simulink model "lateral_autopilot_2e"  (R2018b)
settings: Solver=VariableStepAuto  StartTime=0.0  StopTime=500  RelTol=1e-3
values from neighbouring files (symbols this model uses):
  A = [ ... (first row only)    [lateral_autopilot_2f_params.m]
  B = [0 0 0 0 7.5]'    [lateral_autopilot_2f_params.m]
  C = [eye(4) zeros(4,1)]    [lateral_autopilot_2f_params.m]
  d = 1.5    [lateral_autopilot_2d_params.m]    (also in lateral_autopilot_2f_params.m)
  g = 9.81    [lateral_autopilot_2d_params.m]    (also in lateral_autopilot_2f_params.m)
  kd_phi = (2*zeta_phi*omega_n_phi-a_phi_1)/a_phi_2    [lateral_autopilot_2d_params.m]    (also in lateral_autopilot_2f_params.m)
  ki_chi = omega_chi_phi^2*vg/g    [lateral_autopilot_2d_params.m]    (also in lateral_autopilot_2f_params.m)
  kp_chi = 2*zeta_chi*omega_chi_phi*vg/g    [lateral_autopilot_2d_params.m]    (also in lateral_autopilot_2f_params.m)
  kp_phi = (aileron_max/error_max)*sign(a_phi_2)    [lateral_autopilot_2d_params.m]    (also in lateral_autopilot_2f_params.m)
  vg = 580*km_h2m_s    (= 161.111111111)    [lateral_autopilot_2d_params.m]    (also in lateral_autopilot_2f_params.m)
libraries: simulink_extras x3, simulink x1
settings Model: Creator=dino  LastModifiedBy=dino

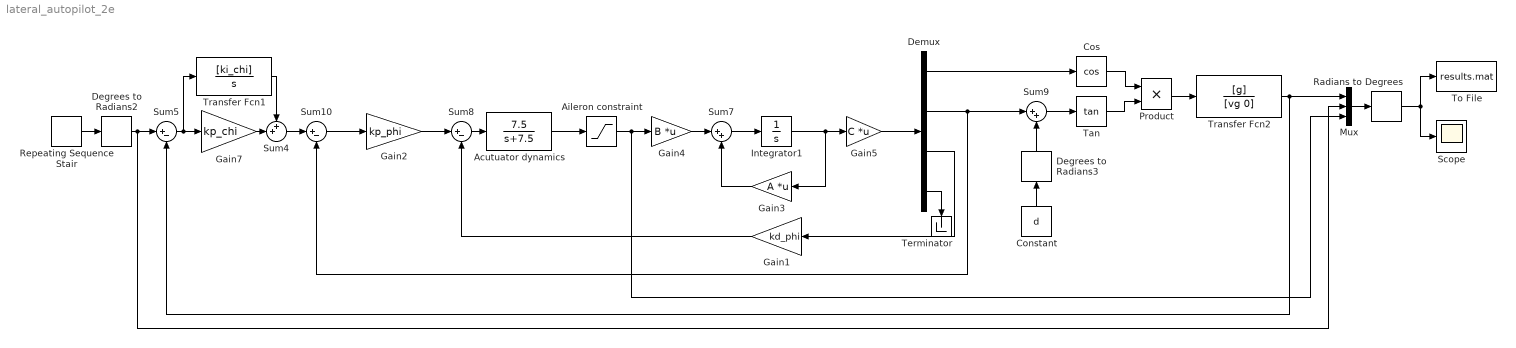
== system lateral_autopilot_2e ==
  Acutuator dynamics : TransferFcn  Numerator=[0 7.5]  Denominator=[1 7.5]
  "Aileron constraint " : Saturate  UpperLimit=30*deg2rad  LowerLimit=-30*deg2rad
  Constant : Constant  Value=d
  Cos : Trigonometry  Operator=cos
  Degrees to Radians2 : simulink_extras/Transformations/Degrees to Radians
  Degrees to Radians3 : simulink_extras/Transformations/Degrees to Radians
  Demux : Demux
  Gain1 : Gain  Gain=kd_phi
  Gain2 : Gain  Gain=kp_phi
  Gain3 : Gain  Gain=A  Multiplication=Matrix(K*u)
  Gain4 : Gain  Gain=B  Multiplication=Matrix(K*u)
  Gain5 : Gain  Gain=C  Multiplication=Matrix(K*u)
  Gain7 : Gain  Gain=kp_chi
  Integrator1 : Integrator
  Mux : Mux  Inputs=3
  Product : Product
  Radians to Degrees : simulink_extras/Transformations/Radians to Degrees
  Repeating Sequence Stair : simulink/Sources/Repeating Sequence Stair  OutValues=step_series.'  tsamp=60  OutMin=[]  OutMax=[]  OutDataTypeStr=double  OutputDataTypeScalingMode=double  OutDataType=fixdt(0,8)  ConRadixGroup=Best Precision: Vector-wise  OutScaling=2^-12
  Scope : Scope
  Sum10 : Sum  Inputs=|+-
  Sum4 : Sum  Inputs=++|
  Sum5 : Sum  Inputs=|+-
  Sum7 : Sum  Inputs=|++
  Sum8 : Sum  Inputs=|+-
  Sum9 : Sum  Inputs=|++
  Tan : Trigonometry  Operator=tan
  Terminator : Terminator
  To File : ToFile  Filename=results.mat
  Transfer Fcn1 : TransferFcn  Numerator=[ki_chi]  Denominator=[1 0]
  Transfer Fcn2 : TransferFcn  Numerator=[g]  Denominator=[vg 0]
  wires:
  Integrator1/1 -> Gain3/1, Gain5/1
  Sum7/1 -> Integrator1/1
  Gain3/1 -> Sum7/2
  Gain2/1 -> Sum8/1
  Gain1/1 -> Sum8/2
  Gain5/1 -> Demux/1
  Demux/3 -> Gain1/1
  Sum9/1 -> Tan/1
  Demux/1 -> Cos/1
  Product/1 -> Transfer Fcn2/1
  Tan/1 -> Product/2
  Cos/1 -> Product/1
  Demux/2 -> Sum10/2, Sum9/1
  Degrees to Radians3/1 -> Sum9/2
  Repeating Sequence Stair/1 -> Degrees to Radians2/1
  Sum5/1 -> Transfer Fcn1/1, Gain7/1
  Sum4/1 -> Sum10/1
  Sum10/1 -> Gain2/1
  Gain4/1 -> Sum7/1
  Degrees to Radians2/1 -> Mux/2, Sum5/1
  Transfer Fcn1/1 -> Sum4/1
  Gain7/1 -> Sum4/2
  Acutuator dynamics/1 -> "Aileron constraint "/1
  Sum8/1 -> Acutuator dynamics/1
  "Aileron constraint "/1 -> Mux/3, Gain4/1
  Constant/1 -> Degrees to Radians3/1
  Demux/4 -> Terminator/1
  Radians to Degrees/1 -> Scope/1, To File/1
  Transfer Fcn2/1 -> Sum5/2, Mux/1
  Mux/1 -> Radians to Degrees/1
